simulink model "PMSM_ROM_NSS_CodeGeneration"  (R2025b)
settings: Solver=FixedStepDiscrete  StartTime=0  StopTime=inf  FixedStep=0.5  RelTol=1e-3
PreLoadFcn:
  | % Load the trained NSS Model
  | load Models/NSSTrainingOutput.mat
  | 
  | % Extract the corresponding input normalizations
  | meanX_nss = NSStrainingOutput.Normalization.Mu{1,1:7};
  | stdX_nss = NSStrainingOutput.Normalization.Sigma{1,1:7};
  | 
  | % Extract output normalization
  | meanY_nss = NSStrainingOutput.Normalization.Mu{1,8:11};
  | stdY_nss = NSStrainingOutput.Normalization.Sigma{1,8:11};
model workspace (MAT data in the model file):
  time = -1
values from neighbouring files (symbols this model uses):
  NSStrainingOutput =     [NSSTrainingOutput.mat]
libraries: slident x1
settings Model: Creator=skeshavm
settings SolverCC: AlgebraicLoopSolver=TrustRegion
settings DataIOCC: SaveFormat=StructureWithTime  SaveOutput=off  SignalLogging=off  DSMLogging=off  SaveTime=off
settings OptimizationCC: DefaultParameterBehavior=Inlined  UseDivisionForNetSlopeComputation=on  GainParamInheritBuiltInType=on  UseFloatMulNetSlope=on  InlineInvariantSignals=on  PassReuseOutputArgsAs=Individual arguments  ZeroExternalMemoryAtStartup=off  ZeroInternalMemoryAtStartup=off  NoFixptDivByZeroProtection=on  EfficientFloat2IntCast=on  LifeSpan=1  OptimizeBlockOrder=speed  DifferentSizesBufferReuse=on  EfficientTunableParamExpr=on
settings DebuggingCC: InheritedTsInSrcMsg=none  MultiTaskCondExecSysMsg=none  MultiTaskRateTransMsg=warning  ParameterTunabilityLossMsg=error  UnconnectedInputMsg=warning  UnconnectedOutputMsg=warning  UnconnectedLineMsg=warning
settings HardwareCC: ProdBitPerPointer=32.0  ProdBitPerSizeT=32.0  ProdBitPerPtrDiffT=32.0  ProdWordSize=32.0  ProdLongLongMode=on  ProdHWDeviceType=Intel->x86-32 (Windows32)  TargetLongLongMode=on
settings ModelReferenceCC: EnableRefExpFcnMdlSchedulingChecks=on
settings SFSimCC: MATLABDynamicMemAlloc=off
settings RTWCC: SystemTargetFile=ert.tlc  TemplateMakefile=ert_default_tmf  BuildConfiguration=Faster Runs  CodeExecutionProfiling=on  GenerateCodeMetricsReport=on  GPUErrorChecks=on  GPUComputeCapability=7.5  DLArmComputeVersion=19.05  Description=Embedded Coder
settings CodeAppCC: ForceParamTrailComments=on  IgnoreCustomStorageClasses=off  OperatorAnnotations=on  SimulinkDataObjDesc=on  SFDataObjDesc=on  CustomSymbolStrGlobalVar=rt$N$M  CustomSymbolStrType=$N$M  CustomSymbolStrFcn=$N$M$F  CustomSymbolStrMacro=$N$M  InsertBlockDesc=on
settings ERTTargetCC: ERTCustomFileTemplate=example_file_process.tlc  ERTFilePackagingFormat=CompactWithDataFile  TargetLangStandard=C99 (ISO)  GenerateSampleERTMain=on  IncludeMdlTerminateFcn=off  CombineSignalStateStructs=on  SuppressErrorStatus=on  SupportAbsoluteTime=off  SupportComplex=off

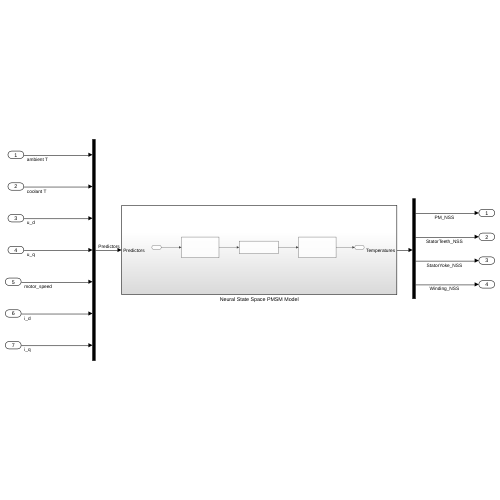
[thumbnail: Simulink's stored preview of the top-level diagram]
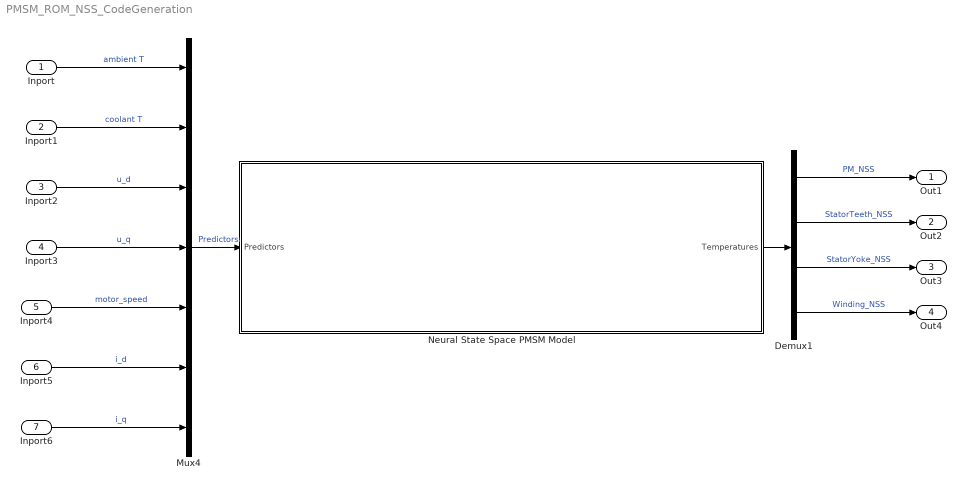
== system PMSM_ROM_NSS_CodeGeneration ==
  Inport : Inport
  Inport1 : Inport  Port=2
  Inport2 : Inport  Port=3
  Inport3 : Inport  Port=4
  Inport4 : Inport  Port=5
  Inport5 : Inport  Port=6
  Inport6 : Inport  Port=7
  Demux1 : Demux
  Mux4 : Mux  Inputs=7
  Neural State Space PMSM Model : Subsystem
  Out1 : Outport
  Out2 : Outport  Port=2
  Out3 : Outport  Port=3
  Out4 : Outport  Port=4
  wires:
  Inport/1 -> Mux4/1  "ambient T"
  Inport1/1 -> Mux4/2  "coolant T"
  Inport2/1 -> Mux4/3  "u_d"
  Inport3/1 -> Mux4/4  "u_q"
  Inport4/1 -> Mux4/5  "motor_speed"
  Inport5/1 -> Mux4/6  "i_d"
  Inport6/1 -> Mux4/7  "i_q"
  Demux1/1 -> Out1/1  "PM_NSS"
  Demux1/2 -> Out2/1  "StatorTeeth_NSS"
  Demux1/3 -> Out3/1  "StatorYoke_NSS"
  Demux1/4 -> Out4/1  "Winding_NSS"
  Mux4/1 -> Neural State Space PMSM Model/1(Predictors)  "Predictors"
  Neural State Space PMSM Model/1(Temperatures) -> Demux1/1

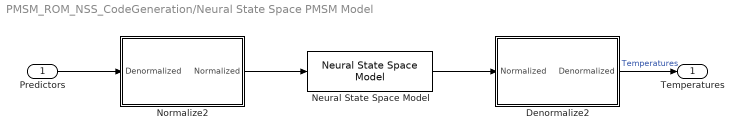
== system PMSM_ROM_NSS_CodeGeneration/Neural State Space PMSM Model ==
  Predictors : Inport
  Denormalize2 : Subsystem
  Neural State Space Model : slident/Models/Neural State Space Model  sys=NSStrainingOutput.NSSModel  x0type=internal  ic=[-1.4912 -1.0704 -1.2954 -1.3511]  returnx=off  returndx=off
  Normalize2 : Subsystem
  Temperatures : Outport
  wires:
  Predictors/1 -> Normalize2/1(Denormalized)
  Neural State Space Model/1 -> Denormalize2/1(Normalized)
  Denormalize2/1(Denormalized) -> Temperatures/1  "Temperatures"
  Normalize2/1(Normalized) -> Neural State Space Model/1

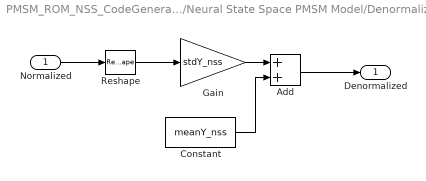
== system PMSM_ROM_NSS_CodeGeneration/Neural State Space PMSM Model/Denormalize2 ==
  Normalized : Inport
  Add : Sum
  Constant : Constant  Value=meanY_nss
  Gain : Gain  Gain=stdY_nss  OutDataTypeStr=single
  Reshape : Reshape
  Denormalized : Outport
  wires:
  Reshape/1 -> Gain/1
  Constant/1 -> Add/2
  Gain/1 -> Add/1
  Add/1 -> Denormalized/1
  Normalized/1 -> Reshape/1

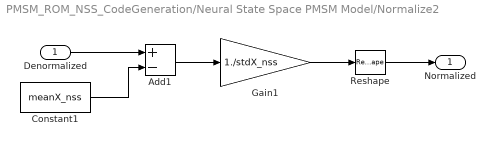
== system PMSM_ROM_NSS_CodeGeneration/Neural State Space PMSM Model/Normalize2 ==
  Denormalized : Inport
  Add1 : Sum  Inputs=+-
  Constant1 : Constant  Value=meanX_nss
  Gain1 : Gain  Gain=1./stdX_nss
  Reshape : Reshape
  Normalized : Outport
  wires:
  Gain1/1 -> Reshape/1
  Add1/1 -> Gain1/1
  Constant1/1 -> Add1/2
  Denormalized/1 -> Add1/1
  Reshape/1 -> Normalized/1
